simulink library "atlas_dynamic_library"  (Simulink 8.4)
settings: Solver=ode45  StartTime=0.0  StopTime=10.0  RelTol=1e-3
values from neighbouring files (symbols this model uses):
  atlas_arm_lr = lr    [atlas_joint_impctrl_sqrt_damping_test_settings_default.m]
  atlas_leg_lr = lr    [atlas_joint_impctrl_sqrt_damping_test_settings_default.m]
  B = d - 0.1*ones(NJL,1)    [atlas_joint_impctrl_sqrt_damping_test_settings_default.m]
  d = 0.2*ones(NJL,1)    [atlas_joint_impctrl_sqrt_damping_test_settings_default.m]
  muC = 8*ones(NJL,1)    [atlas_joint_impctrl_sqrt_damping_test_settings_default.m]
  q0 = q_l    [atlas_joint_impctrl_sqrt_damping_test_settings_default.m]
  qD0 = zeros(1,NJL)'    [atlas_joint_impctrl_sqrt_damping_test_settings_default.m]
  tau_c = muC - 4*ones(NJL,1)    [atlas_joint_impctrl_sqrt_damping_test_settings_default.m]
undefined symbols (not defined in the file or in its folder): atlas_version, delta_s, MPV, qD_s, tau_s
libraries: atlas_dynamic_library x28
settings Model: Creator=schappler  LastModifiedBy=vorndamme

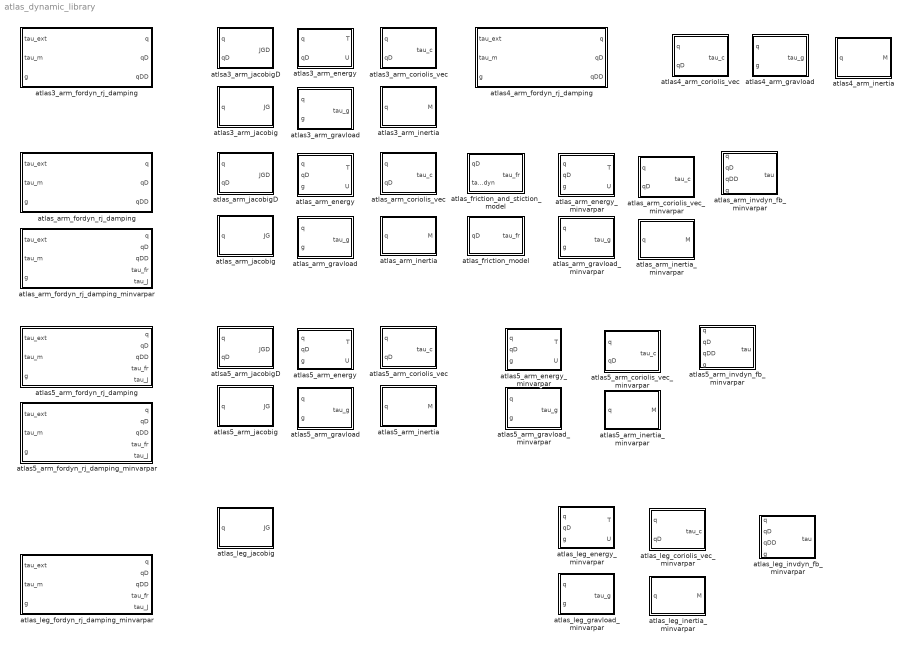
== system atlas_dynamic_library ==
  atlas3_arm_coriolis_vec : Subsystem  TreatAsAtomicUnit=on
  atlas3_arm_energy : Subsystem  TreatAsAtomicUnit=on
  atlas3_arm_fordyn_rj_damping : Subsystem  mask{q0=q0, qD0=qD0, d=d, muC=muC, atlas_arm_lr=atlas_arm_lr}
      mask prompts: q0 "q0 (initial pose)"; qD0 "qD0 (initial velocity)"; d "d (viscous friction)"; muC "muC (coulomb friction)"; atlas_arm_lr "atlas_arm_lr (Arm: left = true, right = false)"
  atlas3_arm_gravload : Subsystem  TreatAsAtomicUnit=on
  atlas3_arm_inertia : Subsystem  TreatAsAtomicUnit=on
  atlas3_arm_jacobig : Subsystem  TreatAsAtomicUnit=on
  atlas4_arm_coriolis_vec : Subsystem  TreatAsAtomicUnit=on
  atlas4_arm_fordyn_rj_damping : Subsystem  mask{q0=q0, qD0=qD0, d=d, muC=muC, atlas_arm_lr=atlas_arm_lr}
      mask prompts: q0 "q0 (initial pose)"; qD0 "qD0 (initial velocity)"; d "d (viscous friction)"; muC "muC (coulomb friction)"; atlas_arm_lr "atlas_arm_lr (Arm: left = true, right = false)"
  atlas4_arm_gravload : Subsystem  TreatAsAtomicUnit=on
  atlas4_arm_inertia : Subsystem  TreatAsAtomicUnit=on
  atlas5_arm_coriolis_vec : Subsystem  TreatAsAtomicUnit=on
  atlas5_arm_coriolis_vec_minvarpar : Subsystem  TreatAsAtomicUnit=on  mask{atlas_arm_lr=atlas_arm_lr, MPV=MPV}
      mask prompts: atlas_arm_lr "atlas_arm_lr (left = true, right = false)"; MPV "MPV (vector of minimal parameters)"
  atlas5_arm_energy : Subsystem  TreatAsAtomicUnit=on
  atlas5_arm_energy_minvarpar : Subsystem  TreatAsAtomicUnit=on  mask{MPV=MPV}
      mask prompts: MPV "MPV (vector of minimal parameters)"
  atlas5_arm_fordyn_rj_damping : Subsystem  mask{q0=q0, qD0=qD0, d=d, muC=muC, atlas_arm_lr=atlas_arm_lr}
      mask prompts: q0 "q0 (initial pose)"; qD0 "qD0 (initial velocity)"; d "d (viscous friction)"; muC "muC (coulomb friction)"; atlas_arm_lr "atlas_arm_lr (Arm: left = true, right = false)"
  atlas5_arm_fordyn_rj_damping_minvarpar : Subsystem  mask{q0=q0, qD0=qD0, d=d, muC=muC, atlas_arm_lr=atlas_arm_lr, MPV=MPV}
      mask prompts: q0 "q0 (initial pose)"; qD0 "qD0 (initial velocity)"; d "d (viscous friction)"; muC "muC (coulomb friction)"; atlas_arm_lr "atlas_arm_lr (Arm: left = true, right = false)"; MPV "MPV (minimal parameter vector)"
  atlas5_arm_gravload : Subsystem  TreatAsAtomicUnit=on
  atlas5_arm_gravload_minvarpar : Subsystem  TreatAsAtomicUnit=on  mask{atlas_arm_lr=atlas_arm_lr, MPV=MPV}
      mask prompts: atlas_arm_lr "atlas_arm_lr (left = true, right = false)"; MPV "MPV (vector of minimal parameters)"
  atlas5_arm_inertia : Subsystem  TreatAsAtomicUnit=on
  atlas5_arm_inertia_minvarpar : Subsystem  TreatAsAtomicUnit=on  mask{atlas_arm_lr=atlas_arm_lr, MPV=MPV}
      mask prompts: atlas_arm_lr "atlas_arm_lr (left = true, right = false)"; MPV "MPV (vector of minimal parameters)"
  atlas5_arm_invdyn_fb_minvarpar : Subsystem  TreatAsAtomicUnit=on  mask{MPV=MPV}
      mask prompts: MPV "MPV (vector of minimal parameters)"
  atlas5_arm_jacobig : Subsystem  TreatAsAtomicUnit=on
  atlas_arm_coriolis_vec : Subsystem  TreatAsAtomicUnit=on
  atlas_arm_coriolis_vec_minvarpar : Subsystem  TreatAsAtomicUnit=on  mask{atlas_arm_lr=atlas_arm_lr, atlas_version=atlas_version, MPV=MPV}
      mask prompts: atlas_arm_lr "atlas_arm_lr (left = true, right = false)"; atlas_version "atlas_version (3, 4)"; MPV "MPV (vecotr of minimal parameters)"
  atlas_arm_energy : Subsystem  TreatAsAtomicUnit=on
  atlas_arm_energy_minvarpar : Subsystem  TreatAsAtomicUnit=on  mask{MPV=MPV}
      mask prompts: MPV "MPV (vector of minimal parameters)"
  atlas_arm_fordyn_rj_damping : Subsystem  mask{q0=q0, qD0=qD0, d=d, muC=muC, atlas_arm_lr=atlas_arm_lr, atlas_version=atlas_version}
      mask prompts: q0 "q0 (initial pose)"; qD0 "qD0 (initial velocity)"; d "d (viscous friction)"; muC "muC (coulomb friction)"; atlas_arm_lr "atlas_arm_lr (Arm: left = true, right = false)"; atlas_version "atlas_version (3, 4)"
  atlas_arm_fordyn_rj_damping_minvarpar : Subsystem  mask{q0=q0, qD0=qD0, d=d, muC=muC, atlas_arm_lr=atlas_arm_lr, atlas_version=atlas_version, MPV=MPV}
      mask prompts: q0 "q0 (initial pose)"; qD0 "qD0 (initial velocity)"; d "d (viscous friction)"; muC "muC (coulomb friction)"; atlas_arm_lr "atlas_arm_lr (Arm: left = true, right = false)"; atlas_version "atlas_version (3, 4)"; MPV "MPV (minimal parameter vector)"
  atlas_arm_gravload : Subsystem  TreatAsAtomicUnit=on
  atlas_arm_gravload_minvarpar : Subsystem  TreatAsAtomicUnit=on  mask{atlas_arm_lr=atlas_arm_lr, atlas_version=atlas_version, MPV=MPV}
      mask prompts: atlas_arm_lr "atlas_arm_lr (left = true, right = false)"; atlas_version "atlas_version (3, 4)"; MPV "MPV (vector of minimal parameters)"
  atlas_arm_inertia : Subsystem  TreatAsAtomicUnit=on
  atlas_arm_inertia_minvarpar : Subsystem  TreatAsAtomicUnit=on  mask{atlas_arm_lr=atlas_arm_lr, atlas_version=atlas_version, MPV=MPV}
      mask prompts: atlas_arm_lr "atlas_arm_lr (left = true, right = false)"; atlas_version "atlas_version (3, 4)"; MPV "MPV (vector of minimal parameters)"
  atlas_arm_invdyn_fb_minvarpar : Subsystem  TreatAsAtomicUnit=on  mask{MPV=MPV}
      mask prompts: MPV "MPV (vector of minimal parameters)"
  atlas_arm_jacobig : Subsystem  TreatAsAtomicUnit=on
  atlas_arm_jacobigD : Subsystem  TreatAsAtomicUnit=on
  atlas_friction_and_stiction_model : Subsystem  TreatAsAtomicUnit=on  mask{tau_c=tau_c, B=B, tau_s=tau_s, qD_s=qD_s, delta_s=delta_s}
      mask prompts: tau_c "tau_c (vector with coulomb friciton momentums for all joints)"; B "B (vector with viscous friction coefficients of all joints)"; tau_s "tau_s (vector with sticition momentums of all joints)"; qD_s "qD_s (vector with Stribeck velocities of all joints)"; delta_s "delta_s (vector with stiction exponents for all joints)"
  atlas_friction_model : Subsystem  TreatAsAtomicUnit=on  mask{muC=muC, d=d}
  atlas_leg_coriolis_vec_minvarpar : Subsystem  TreatAsAtomicUnit=on  mask{atlas_arm_lr=atlas_leg_lr, atlas_version=atlas_version, MPV=MPV}
      mask prompts: atlas_arm_lr "atlas_arm_lr (left = true, right = false)"; atlas_version "atlas_version (3, 4)"; MPV "MPV (vecotr of minimal parameters)"
  atlas_leg_energy_minvarpar : Subsystem  TreatAsAtomicUnit=on  mask{MPV=MPV, atlas_version=atlas_version}
      mask prompts: MPV "MPV (vector of minimal parameters)"; atlas_version "Version"
  atlas_leg_fordyn_rj_damping_minvarpar : Subsystem  mask{q0=q0, qD0=qD0, d=d, muC=muC, atlas_arm_lr=atlas_leg_lr, atlas_version=uint8(5), MPV=MPV}
      mask prompts: q0 "q0 (initial pose)"; qD0 "qD0 (initial velocity)"; d "d (viscous friction)"; muC "muC (coulomb friction)"; atlas_arm_lr "atlas_leg_lr (Leg: left = true, right = false)"; atlas_version "atlas_version (3, 4)"; MPV "MPV (minimal parameter vector)"
  atlas_leg_gravload_minvarpar : Subsystem  TreatAsAtomicUnit=on  mask{atlas_arm_lr=atlas_leg_lr, atlas_version=atlas_version, MPV=MPV}
      mask prompts: atlas_arm_lr "atlas_arm_lr (left = true, right = false)"; atlas_version "atlas_version (3, 4)"; MPV "MPV (vector of minimal parameters)"
  atlas_leg_inertia_minvarpar : Subsystem  TreatAsAtomicUnit=on  mask{atlas_arm_lr=atlas_leg_lr, atlas_version=atlas_version, MPV=MPV}
      mask prompts: atlas_arm_lr "atlas_arm_lr (left = true, right = false)"; atlas_version "atlas_version (3, 4)"; MPV "MPV (vector of minimal parameters)"
  atlas_leg_invdyn_fb_minvarpar : Subsystem  TreatAsAtomicUnit=on  mask{MPV=MPV}
      mask prompts: MPV "MPV (vector of minimal parameters)"
  atlas_leg_jacobig : Subsystem  TreatAsAtomicUnit=on  mask{atlas_version=atlas_version, atlas_leg_lr=atlas_leg_lr}
      mask prompts: atlas_version "Version"; atlas_leg_lr "LeftRight"
  atlsa3_arm_jacobigD : Subsystem  TreatAsAtomicUnit=on
  atlsa5_arm_jacobigD : Subsystem  TreatAsAtomicUnit=on

== system atlas_dynamic_library/atlas3_arm_coriolis_vec ==
  q : Inport
  qD : Inport  Port=2
  mFcn_c : MATLAB Function  TreatAsAtomicUnit=on
  tau_c : Outport
  wires:
  mFcn_c/1(tau_c) -> tau_c/1
  qD/1 -> mFcn_c/2(qD)
  q/1 -> mFcn_c/1(q)

== system atlas_dynamic_library/atlas3_arm_energy ==
  q : Inport
  qD : Inport  Port=2
  atlas3_arm_energy_fb : MATLAB Function  TreatAsAtomicUnit=on  mask{edit_lr=atlas_arm_lr}
      mask prompts: edit_lr "Arm (left = true, right = false)"
      mask init:
      | if edit_lr == 1
      |   atlas_arm_lr = true; % left
      | else
      |   atlas_arm_lr = false; % right
      | end
  T : Outport
  U : Outport  Port=2
  wires:
  q/1 -> atlas3_arm_energy_fb/1(q)
  qD/1 -> atlas3_arm_energy_fb/2(qD)
  atlas3_arm_energy_fb/2(U) -> U/1
  atlas3_arm_energy_fb/1(T) -> T/1

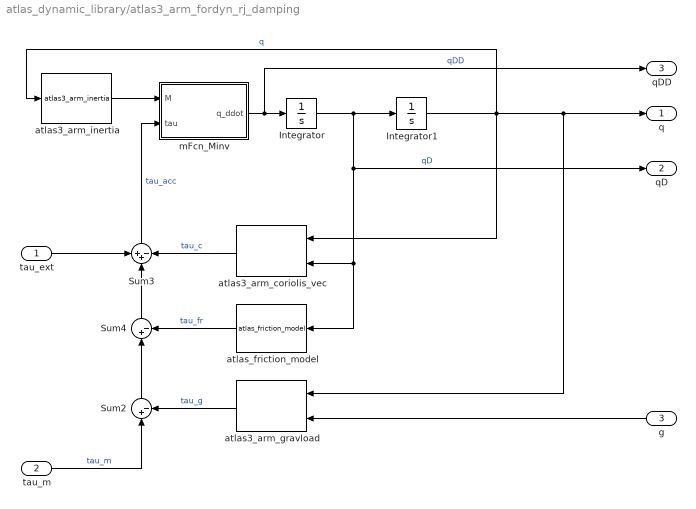
== system atlas_dynamic_library/atlas3_arm_fordyn_rj_damping ==
  "tau_ext " : Inport
  tau_m : Inport  Port=2
  g : Inport  Port=3
  Integrator : Integrator  InitialCondition=qD0
  Integrator1 : Integrator  InitialCondition=q0
  Sum2 : Sum  Inputs=|+-
  Sum3 : Sum  Inputs=++-
  Sum4 : Sum  Inputs=|+-
  atlas3_arm_coriolis_vec : atlas_dynamic_library/atlas3_arm_coriolis_vec
  atlas3_arm_gravload : atlas_dynamic_library/atlas3_arm_gravload
  atlas3_arm_inertia : atlas_dynamic_library/atlas3_arm_inertia
  atlas_friction_model : atlas_dynamic_library/atlas_friction_model  muC=muC  d=d
  mFcn_Minv : MATLAB Function  TreatAsAtomicUnit=on
  q : Outport
  qD : Outport  Port=2
  qDD : Outport  Port=3
  wires:
  atlas3_arm_gravload/1 -> Sum2/2  "tau_g"
  Integrator1/1 -> atlas3_arm_inertia/1, atlas3_arm_coriolis_vec/1, atlas3_arm_gravload/1, q/1  "q"
  Sum2/1 -> Sum4/1
  mFcn_Minv/1(q_ddot) -> qDD/1, Integrator/1  "qDD"
  Sum4/1 -> Sum3/2
  atlas3_arm_coriolis_vec/1 -> Sum3/3  "tau_c"
  atlas_friction_model/1 -> Sum4/2  "tau_fr"
  "tau_ext "/1 -> Sum3/1
  tau_m/1 -> Sum2/1  "tau_m"
  Integrator/1 -> qD/1, atlas_friction_model/1, atlas3_arm_coriolis_vec/2, Integrator1/1  "qD"
  Sum3/1 -> mFcn_Minv/2(tau)  "tau_acc"
  atlas3_arm_inertia/1 -> mFcn_Minv/1(M)
  g/1 -> atlas3_arm_gravload/2

== system atlas_dynamic_library/atlas3_arm_gravload ==
  q : Inport
  g : Inport  Port=2
  mFcn_g : MATLAB Function  TreatAsAtomicUnit=on
  tau_g : Outport
  wires:
  q/1 -> mFcn_g/1(q)
  mFcn_g/1(tau_g) -> tau_g/1
  g/1 -> mFcn_g/2(g)

== system atlas_dynamic_library/atlas3_arm_inertia ==
  q : Inport
  mFcn_M : MATLAB Function  TreatAsAtomicUnit=on
  M : Outport
  wires:
  q/1 -> mFcn_M/1(q)
  mFcn_M/1(M) -> M/1

== system atlas_dynamic_library/atlas3_arm_jacobig ==
  q : Inport
  atlas3_arm_jacobig : MATLAB Function  TreatAsAtomicUnit=on  mask{edit_lr=atlas_arm_lr}
      mask prompts: edit_lr "Arm (left = true, right = false)"
      mask init:
      | if edit_lr == 1
      |   atlas_arm_lr = true; % left
      | else
      |   atlas_arm_lr = false; % right
      | end
  JG : Outport
  wires:
  atlas3_arm_jacobig/1(JG) -> JG/1
  q/1 -> atlas3_arm_jacobig/1(q)

== system atlas_dynamic_library/atlas4_arm_coriolis_vec ==
  q : Inport
  qD : Inport  Port=2
  mFcn_c : MATLAB Function  TreatAsAtomicUnit=on
  tau_c : Outport
  wires:
  mFcn_c/1(tau_c) -> tau_c/1
  q/1 -> mFcn_c/1(q)
  qD/1 -> mFcn_c/2(qD)

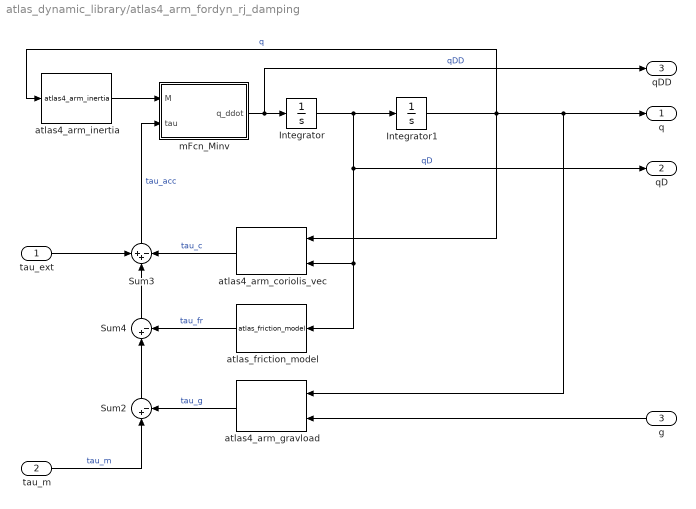
== system atlas_dynamic_library/atlas4_arm_fordyn_rj_damping ==
  "tau_ext " : Inport
  tau_m : Inport  Port=2
  g : Inport  Port=3
  Integrator : Integrator  InitialCondition=qD0
  Integrator1 : Integrator  InitialCondition=q0
  Sum2 : Sum  Inputs=|+-
  Sum3 : Sum  Inputs=++-
  Sum4 : Sum  Inputs=|+-
  atlas4_arm_coriolis_vec : atlas_dynamic_library/atlas4_arm_coriolis_vec
  atlas4_arm_gravload : atlas_dynamic_library/atlas4_arm_gravload
  atlas4_arm_inertia : atlas_dynamic_library/atlas4_arm_inertia
  atlas_friction_model : atlas_dynamic_library/atlas_friction_model  muC=muC  d=d
  mFcn_Minv : MATLAB Function  TreatAsAtomicUnit=on
  q : Outport
  qD : Outport  Port=2
  qDD : Outport  Port=3
  wires:
  atlas4_arm_gravload/1 -> Sum2/2  "tau_g"
  Integrator1/1 -> atlas4_arm_inertia/1, atlas4_arm_coriolis_vec/1, atlas4_arm_gravload/1, q/1  "q"
  Sum2/1 -> Sum4/1
  mFcn_Minv/1(q_ddot) -> qDD/1, Integrator/1  "qDD"
  Sum4/1 -> Sum3/2
  atlas4_arm_coriolis_vec/1 -> Sum3/3  "tau_c"
  atlas_friction_model/1 -> Sum4/2  "tau_fr"
  "tau_ext "/1 -> Sum3/1
  tau_m/1 -> Sum2/1  "tau_m"
  Integrator/1 -> qD/1, atlas_friction_model/1, atlas4_arm_coriolis_vec/2, Integrator1/1  "qD"
  Sum3/1 -> mFcn_Minv/2(tau)  "tau_acc"
  atlas4_arm_inertia/1 -> mFcn_Minv/1(M)
  g/1 -> atlas4_arm_gravload/2

== system atlas_dynamic_library/atlas4_arm_gravload ==
  q : Inport
  g : Inport  Port=2
  mFcn_g : MATLAB Function  TreatAsAtomicUnit=on
  tau_g : Outport
  wires:
  mFcn_g/1(tau_g) -> tau_g/1
  q/1 -> mFcn_g/1(q)
  g/1 -> mFcn_g/2(g)

== system atlas_dynamic_library/atlas4_arm_inertia ==
  q : Inport
  mFcn_M : MATLAB Function  TreatAsAtomicUnit=on
  M : Outport
  wires:
  q/1 -> mFcn_M/1(q)
  mFcn_M/1(M) -> M/1

== system atlas_dynamic_library/atlas5_arm_coriolis_vec ==
  q : Inport
  qD : Inport  Port=2
  mFcn_c : MATLAB Function  TreatAsAtomicUnit=on
  tau_c : Outport
  wires:
  mFcn_c/1(tau_c) -> tau_c/1
  qD/1 -> mFcn_c/2(qD)
  q/1 -> mFcn_c/1(q)

== system atlas_dynamic_library/atlas5_arm_coriolis_vec_minvarpar ==
  q : Inport
  qD : Inport  Port=2
  mFcn_c : MATLAB Function  TreatAsAtomicUnit=on
  tau_c : Outport
  wires:
  qD/1 -> mFcn_c/2(qD)
  q/1 -> mFcn_c/1(q)
  mFcn_c/1(tau_c) -> tau_c/1

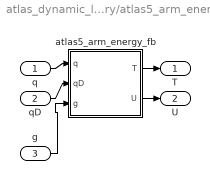
== system atlas_dynamic_library/atlas5_arm_energy ==
  q : Inport
  qD : Inport  Port=2
  g : Inport  Port=3
  atlas5_arm_energy_fb : MATLAB Function  TreatAsAtomicUnit=on  mask{edit_lr=atlas_arm_lr}
      mask prompts: edit_lr "Arm (left = true, right = false)"
      mask init:
      | if edit_lr == 1
      |   atlas_arm_lr = true; % left
      | else
      |   atlas_arm_lr = false; % right
      | end
  T : Outport
  U : Outport  Port=2
  wires:
  q/1 -> atlas5_arm_energy_fb/1(q)
  qD/1 -> atlas5_arm_energy_fb/2(qD)
  atlas5_arm_energy_fb/2(U) -> U/1
  atlas5_arm_energy_fb/1(T) -> T/1
  g/1 -> atlas5_arm_energy_fb/3(g)

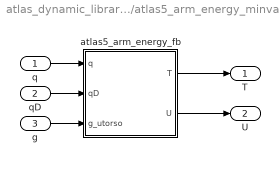
== system atlas_dynamic_library/atlas5_arm_energy_minvarpar ==
  q : Inport
  qD : Inport  Port=2
  g : Inport  Port=3
  atlas5_arm_energy_fb : MATLAB Function  TreatAsAtomicUnit=on
  T : Outport
  U : Outport  Port=2
  wires:
  g/1 -> atlas5_arm_energy_fb/3(g_utorso)
  q/1 -> atlas5_arm_energy_fb/1(q)
  atlas5_arm_energy_fb/2(U) -> U/1
  atlas5_arm_energy_fb/1(T) -> T/1
  qD/1 -> atlas5_arm_energy_fb/2(qD)

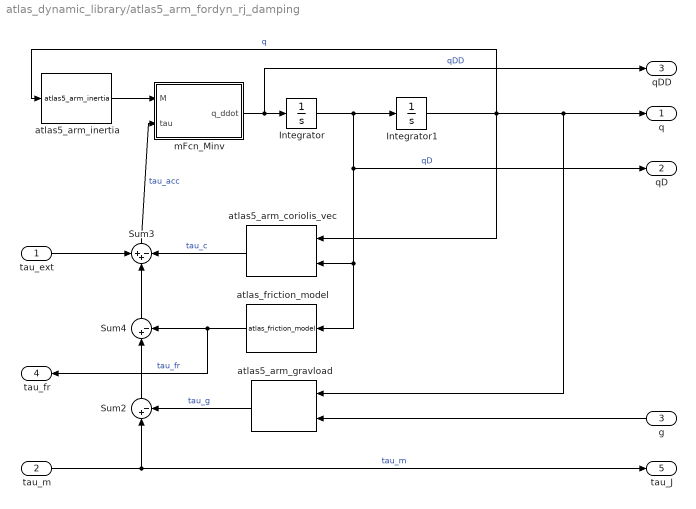
== system atlas_dynamic_library/atlas5_arm_fordyn_rj_damping ==
  "tau_ext " : Inport
  tau_m : Inport  Port=2
  g : Inport  Port=3
  Integrator : Integrator  InitialCondition=qD0
  Integrator1 : Integrator  InitialCondition=q0
  Sum2 : Sum  Inputs=|+-
  Sum3 : Sum  Inputs=++-
  Sum4 : Sum  Inputs=|+-
  atlas5_arm_coriolis_vec : atlas_dynamic_library/atlas5_arm_coriolis_vec
  atlas5_arm_gravload : atlas_dynamic_library/atlas5_arm_gravload
  atlas5_arm_inertia : atlas_dynamic_library/atlas5_arm_inertia
  atlas_friction_model : atlas_dynamic_library/atlas_friction_model  muC=muC  d=d
  mFcn_Minv : MATLAB Function  TreatAsAtomicUnit=on
  q : Outport
  qD : Outport  Port=2
  qDD : Outport  Port=3
  tau_fr : Outport  Port=4
  tau_J : Outport  Port=5
  wires:
  atlas5_arm_gravload/1 -> Sum2/2  "tau_g"
  Integrator1/1 -> atlas5_arm_inertia/1, atlas5_arm_coriolis_vec/1, atlas5_arm_gravload/1, q/1  "q"
  Sum2/1 -> Sum4/1
  mFcn_Minv/1(q_ddot) -> qDD/1, Integrator/1  "qDD"
  Sum4/1 -> Sum3/2
  atlas5_arm_coriolis_vec/1 -> Sum3/3  "tau_c"
  atlas_friction_model/1 -> tau_fr/1, Sum4/2  "tau_fr"
  "tau_ext "/1 -> Sum3/1
  Integrator/1 -> qD/1, atlas5_arm_coriolis_vec/2, atlas_friction_model/1, Integrator1/1  "qD"
  Sum3/1 -> mFcn_Minv/2(tau)  "tau_acc"
  atlas5_arm_inertia/1 -> mFcn_Minv/1(M)
  g/1 -> atlas5_arm_gravload/2
  tau_m/1 -> Sum2/1, tau_J/1  "tau_m"

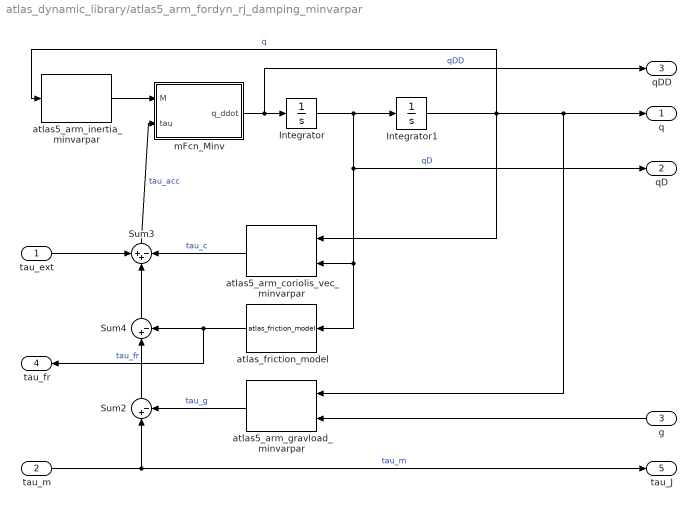
== system atlas_dynamic_library/atlas5_arm_fordyn_rj_damping_minvarpar ==
  "tau_ext " : Inport
  tau_m : Inport  Port=2
  g : Inport  Port=3
  Integrator : Integrator  InitialCondition=qD0
  Integrator1 : Integrator  InitialCondition=q0
  Sum2 : Sum  Inputs=|+-
  Sum3 : Sum  Inputs=++-
  Sum4 : Sum  Inputs=|+-
  atlas5_arm_coriolis_vec_minvarpar : atlas_dynamic_library/atlas5_arm_coriolis_vec_minvarpar
  atlas5_arm_gravload_minvarpar : atlas_dynamic_library/atlas5_arm_gravload_minvarpar
  atlas5_arm_inertia_minvarpar : atlas_dynamic_library/atlas5_arm_inertia_minvarpar
  atlas_friction_model : atlas_dynamic_library/atlas_friction_model  muC=muC  d=d
  mFcn_Minv : MATLAB Function  TreatAsAtomicUnit=on
  q : Outport
  qD : Outport  Port=2
  qDD : Outport  Port=3
  tau_fr : Outport  Port=4
  tau_J : Outport  Port=5
  wires:
  atlas5_arm_gravload_minvarpar/1 -> Sum2/2  "tau_g"
  Integrator1/1 -> atlas5_arm_coriolis_vec_minvarpar/1, atlas5_arm_inertia_minvarpar/1, atlas5_arm_gravload_minvarpar/1, q/1  "q"
  Sum2/1 -> Sum4/1
  mFcn_Minv/1(q_ddot) -> qDD/1, Integrator/1  "qDD"
  Sum4/1 -> Sum3/2
  atlas5_arm_coriolis_vec_minvarpar/1 -> Sum3/3  "tau_c"
  atlas_friction_model/1 -> tau_fr/1, Sum4/2  "tau_fr"
  "tau_ext "/1 -> Sum3/1
  Integrator/1 -> qD/1, atlas5_arm_coriolis_vec_minvarpar/2, atlas_friction_model/1, Integrator1/1  "qD"
  Sum3/1 -> mFcn_Minv/2(tau)  "tau_acc"
  atlas5_arm_inertia_minvarpar/1 -> mFcn_Minv/1(M)
  g/1 -> atlas5_arm_gravload_minvarpar/2
  tau_m/1 -> tau_J/1, Sum2/1  "tau_m"

== system atlas_dynamic_library/atlas5_arm_gravload ==
  q : Inport
  g : Inport  Port=2
  mFcn_g : MATLAB Function  TreatAsAtomicUnit=on
  tau_g : Outport
  wires:
  q/1 -> mFcn_g/1(q)
  mFcn_g/1(tau_g) -> tau_g/1
  g/1 -> mFcn_g/2(g)

== system atlas_dynamic_library/atlas5_arm_gravload_minvarpar ==
  q : Inport
  g : Inport  Port=2
  mFcn_g : MATLAB Function  TreatAsAtomicUnit=on
  tau_g : Outport
  wires:
  g/1 -> mFcn_g/2(g)
  mFcn_g/1(tau_g) -> tau_g/1
  q/1 -> mFcn_g/1(q)

== system atlas_dynamic_library/atlas5_arm_inertia ==
  q : Inport
  mFcn_M : MATLAB Function  TreatAsAtomicUnit=on
  M : Outport
  wires:
  q/1 -> mFcn_M/1(q)
  mFcn_M/1(M) -> M/1

== system atlas_dynamic_library/atlas5_arm_inertia_minvarpar ==
  q : Inport
  mFcn_M : MATLAB Function  TreatAsAtomicUnit=on
  M : Outport
  wires:
  mFcn_M/1(M) -> M/1
  q/1 -> mFcn_M/1(q)

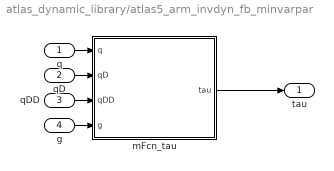
== system atlas_dynamic_library/atlas5_arm_invdyn_fb_minvarpar ==
  q : Inport
  qD : Inport  Port=2
  qDD : Inport  Port=3
  g : Inport  Port=4
  mFcn_tau : MATLAB Function  TreatAsAtomicUnit=on
  tau : Outport
  wires:
  g/1 -> mFcn_tau/4(g)
  qDD/1 -> mFcn_tau/3(qDD)
  qD/1 -> mFcn_tau/2(qD)
  q/1 -> mFcn_tau/1(q)
  mFcn_tau/1(tau) -> tau/1

== system atlas_dynamic_library/atlas5_arm_jacobig ==
  q : Inport
  atlas5_arm_jacobig : MATLAB Function  TreatAsAtomicUnit=on  mask{edit_lr=atlas_arm_lr}
      mask prompts: edit_lr "Arm (left = true, right = false)"
      mask init:
      | if edit_lr == 1
      |   atlas_arm_lr = true; % left
      | else
      |   atlas_arm_lr = false; % right
      | end
  JG : Outport
  wires:
  atlas5_arm_jacobig/1(JG) -> JG/1
  q/1 -> atlas5_arm_jacobig/1(q)

== system atlas_dynamic_library/atlas_arm_coriolis_vec ==
  q : Inport
  qD : Inport  Port=2
  mFcn_c : MATLAB Function  TreatAsAtomicUnit=on
  tau_c : Outport
  wires:
  mFcn_c/1(tau_c) -> tau_c/1
  q/1 -> mFcn_c/1(q)
  qD/1 -> mFcn_c/2(qD)

== system atlas_dynamic_library/atlas_arm_coriolis_vec_minvarpar ==
  q : Inport
  qD : Inport  Port=2
  mFcn_c : MATLAB Function  TreatAsAtomicUnit=on
  tau_c : Outport
  wires:
  qD/1 -> mFcn_c/2(qD)
  q/1 -> mFcn_c/1(q)
  mFcn_c/1(tau_c) -> tau_c/1

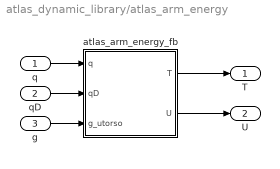
== system atlas_dynamic_library/atlas_arm_energy ==
  q : Inport
  qD : Inport  Port=2
  g : Inport  Port=3
  atlas_arm_energy_fb : MATLAB Function  TreatAsAtomicUnit=on
  T : Outport
  U : Outport  Port=2
  wires:
  qD/1 -> atlas_arm_energy_fb/2(qD)
  atlas_arm_energy_fb/1(T) -> T/1
  atlas_arm_energy_fb/2(U) -> U/1
  q/1 -> atlas_arm_energy_fb/1(q)
  g/1 -> atlas_arm_energy_fb/3(g_utorso)

== system atlas_dynamic_library/atlas_arm_energy_minvarpar ==
  q : Inport
  qD : Inport  Port=2
  g : Inport  Port=3
  atlas_arm_energy_fb : MATLAB Function  TreatAsAtomicUnit=on
  T : Outport
  U : Outport  Port=2
  wires:
  g/1 -> atlas_arm_energy_fb/3(g_utorso)
  q/1 -> atlas_arm_energy_fb/1(q)
  atlas_arm_energy_fb/2(U) -> U/1
  atlas_arm_energy_fb/1(T) -> T/1
  qD/1 -> atlas_arm_energy_fb/2(qD)

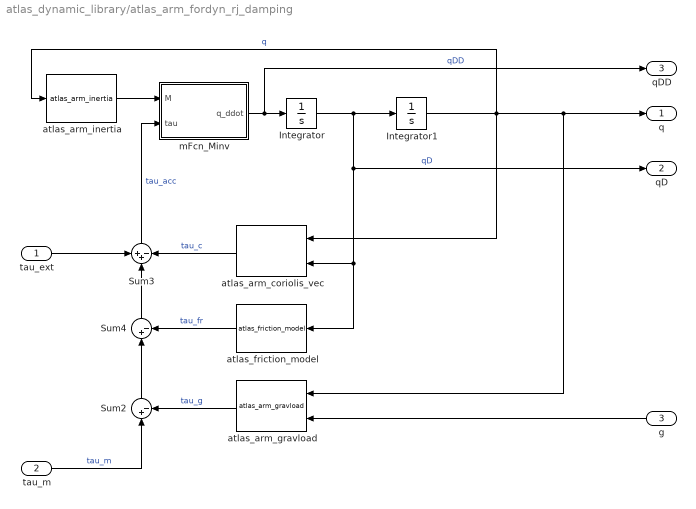
== system atlas_dynamic_library/atlas_arm_fordyn_rj_damping ==
  "tau_ext " : Inport
  tau_m : Inport  Port=2
  g : Inport  Port=3
  Integrator : Integrator  InitialCondition=qD0
  Integrator1 : Integrator  InitialCondition=q0
  Sum2 : Sum  Inputs=|+-
  Sum3 : Sum  Inputs=++-
  Sum4 : Sum  Inputs=|+-
  atlas_arm_coriolis_vec : atlas_dynamic_library/atlas_arm_coriolis_vec
  atlas_arm_gravload : atlas_dynamic_library/atlas_arm_gravload
  atlas_arm_inertia : atlas_dynamic_library/atlas_arm_inertia
  atlas_friction_model : atlas_dynamic_library/atlas_friction_model  muC=muC  d=d
  mFcn_Minv : MATLAB Function  TreatAsAtomicUnit=on
  q : Outport
  qD : Outport  Port=2
  qDD : Outport  Port=3
  wires:
  atlas_arm_gravload/1 -> Sum2/2  "tau_g"
  Integrator1/1 -> atlas_arm_inertia/1, atlas_arm_coriolis_vec/1, atlas_arm_gravload/1, q/1  "q"
  Sum2/1 -> Sum4/1
  mFcn_Minv/1(q_ddot) -> qDD/1, Integrator/1  "qDD"
  Sum4/1 -> Sum3/2
  atlas_arm_coriolis_vec/1 -> Sum3/3  "tau_c"
  atlas_friction_model/1 -> Sum4/2  "tau_fr"
  "tau_ext "/1 -> Sum3/1
  tau_m/1 -> Sum2/1  "tau_m"
  Integrator/1 -> qD/1, atlas_friction_model/1, atlas_arm_coriolis_vec/2, Integrator1/1  "qD"
  Sum3/1 -> mFcn_Minv/2(tau)  "tau_acc"
  atlas_arm_inertia/1 -> mFcn_Minv/1(M)
  g/1 -> atlas_arm_gravload/2

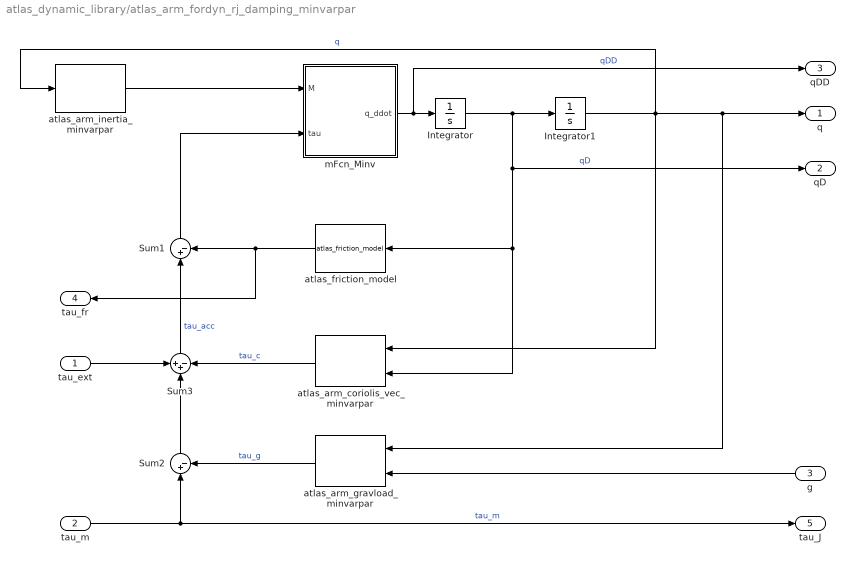
== system atlas_dynamic_library/atlas_arm_fordyn_rj_damping_minvarpar ==
  "tau_ext " : Inport
  tau_m : Inport  Port=2
  g : Inport  Port=3
  Integrator : Integrator  InitialCondition=qD0
  Integrator1 : Integrator  InitialCondition=q0
  Sum1 : Sum  Inputs=|+-
  Sum2 : Sum  Inputs=|+-
  Sum3 : Sum  Inputs=++-
  atlas_arm_coriolis_vec_minvarpar : atlas_dynamic_library/atlas_arm_coriolis_vec_minvarpar  atlas_arm_lr=atlas_arm_lr  atlas_version=atlas_version  MPV=MPV
  atlas_arm_gravload_minvarpar : atlas_dynamic_library/atlas_arm_gravload_minvarpar  atlas_arm_lr=atlas_arm_lr  atlas_version=atlas_version  MPV=MPV
  atlas_arm_inertia_minvarpar : atlas_dynamic_library/atlas_arm_inertia_minvarpar  atlas_arm_lr=atlas_arm_lr  atlas_version=atlas_version  MPV=MPV
  atlas_friction_model : atlas_dynamic_library/atlas_friction_model  muC=muC  d=d
  mFcn_Minv : MATLAB Function  TreatAsAtomicUnit=on
  q : Outport
  qD : Outport  Port=2
  qDD : Outport  Port=3
  tau_fr : Outport  Port=4
  tau_J : Outport  Port=5
  wires:
  atlas_arm_gravload_minvarpar/1 -> Sum2/2  "tau_g"
  Integrator1/1 -> atlas_arm_inertia_minvarpar/1, atlas_arm_coriolis_vec_minvarpar/1, atlas_arm_gravload_minvarpar/1, q/1  "q"
  mFcn_Minv/1(q_ddot) -> qDD/1, Integrator/1  "qDD"
  Sum2/1 -> Sum3/2
  atlas_arm_coriolis_vec_minvarpar/1 -> Sum3/3  "tau_c"
  "tau_ext "/1 -> Sum3/1
  tau_m/1 -> tau_J/1, Sum2/1  "tau_m"
  Integrator/1 -> qD/1, atlas_friction_model/1, atlas_arm_coriolis_vec_minvarpar/2, Integrator1/1  "qD"
  atlas_arm_inertia_minvarpar/1 -> mFcn_Minv/1(M)
  g/1 -> atlas_arm_gravload_minvarpar/2
  Sum3/1 -> Sum1/1  "tau_acc"
  atlas_friction_model/1 -> Sum1/2, tau_fr/1
  Sum1/1 -> mFcn_Minv/2(tau)

== system atlas_dynamic_library/atlas_arm_gravload ==
  q : Inport
  g : Inport  Port=2
  mFcn_g : MATLAB Function  TreatAsAtomicUnit=on
  tau_g : Outport
  wires:
  q/1 -> mFcn_g/1(q)
  mFcn_g/1(tau_g) -> tau_g/1
  g/1 -> mFcn_g/2(g)

== system atlas_dynamic_library/atlas_arm_gravload_minvarpar ==
  q : Inport
  g : Inport  Port=2
  mFcn_g : MATLAB Function  TreatAsAtomicUnit=on
  tau_g : Outport
  wires:
  g/1 -> mFcn_g/2(g)
  mFcn_g/1(tau_g) -> tau_g/1
  q/1 -> mFcn_g/1(q)

== system atlas_dynamic_library/atlas_arm_inertia ==
  q : Inport
  mFcn_M : MATLAB Function  TreatAsAtomicUnit=on
  M : Outport
  wires:
  mFcn_M/1(M) -> M/1
  q/1 -> mFcn_M/1(q)

== system atlas_dynamic_library/atlas_arm_inertia_minvarpar ==
  q : Inport
  mFcn_M : MATLAB Function  TreatAsAtomicUnit=on
  M : Outport
  wires:
  q/1 -> mFcn_M/1(q)
  mFcn_M/1(M) -> M/1

== system atlas_dynamic_library/atlas_arm_invdyn_fb_minvarpar ==
  q : Inport
  qD : Inport  Port=2
  qDD : Inport  Port=3
  g : Inport  Port=4
  mFcn_tau : MATLAB Function  TreatAsAtomicUnit=on
  tau : Outport
  wires:
  mFcn_tau/1(tau) -> tau/1
  q/1 -> mFcn_tau/1(q)
  qD/1 -> mFcn_tau/2(qD)
  qDD/1 -> mFcn_tau/3(qDD)
  g/1 -> mFcn_tau/4(g)

== system atlas_dynamic_library/atlas_arm_jacobig ==
  q : Inport
  atlas_arm_jacobig : MATLAB Function  TreatAsAtomicUnit=on  mask{edit_lr=atlas_arm_lr, edit_version=atlas_version}
      mask prompts: edit_lr "Arm (left = true, right = false)"; edit_version "Version (3, 4)"
      mask init:
      | if edit_lr == 1
      |   atlas_arm_lr = true; % left
      | else
      |   atlas_arm_lr = false; % right
      | end
      | 
      | if edit_version == 3
      |   atlas_version = uint8(3);
      | elseif edit_version == 4
      |   atlas_version = uint8(4);
      | else
      |   error('Version %d not implemented', edit_version);
      | end
  JG : Outport
  wires:
  q/1 -> atlas_arm_jacobig/1(q)
  atlas_arm_jacobig/1(JG) -> JG/1

== system atlas_dynamic_library/atlas_arm_jacobigD ==
  q : Inport
  qD : Inport  Port=2
  atlas_arm_jacobigD : MATLAB Function  TreatAsAtomicUnit=on  mask{edit_lr=atlas_arm_lr, edit_version=atlas_version}
      mask prompts: edit_lr "Arm (left = true, right = false)"; edit_version "Version (3, 4)"
      mask init:
      | if edit_lr == 1
      |   atlas_arm_lr = true; % left
      | else
      |   atlas_arm_lr = false; % right
      | end
  JGD : Outport
  wires:
  qD/1 -> atlas_arm_jacobigD/2(qD)
  q/1 -> atlas_arm_jacobigD/1(q)
  atlas_arm_jacobigD/1(JGD) -> JGD/1

== system atlas_dynamic_library/atlas_friction_and_stiction_model ==
  qD : Inport
  tau_dyn : Inport  Port=2
  atlas_friction_model : MATLAB Function  TreatAsAtomicUnit=on
  tau_fr : Outport
  wires:
  qD/1 -> atlas_friction_model/1(qD)
  atlas_friction_model/1(tau_reib) -> tau_fr/1
  tau_dyn/1 -> atlas_friction_model/2(tau_dyn)

== system atlas_dynamic_library/atlas_friction_model ==
  qD : Inport
  atlas_friction_model : MATLAB Function  TreatAsAtomicUnit=on
  tau_fr : Outport
  wires:
  qD/1 -> atlas_friction_model/1(qD)
  atlas_friction_model/1(tau_fr) -> tau_fr/1

== system atlas_dynamic_library/atlas_leg_coriolis_vec_minvarpar ==
  q : Inport
  qD : Inport  Port=2
  mFcn_c : MATLAB Function  TreatAsAtomicUnit=on
  tau_c : Outport
  wires:
  mFcn_c/1(tau_c) -> tau_c/1
  q/1 -> mFcn_c/1(q)
  qD/1 -> mFcn_c/2(qD)

== system atlas_dynamic_library/atlas_leg_energy_minvarpar ==
  q : Inport
  qD : Inport  Port=2
  g : Inport  Port=3
  atlas_leg_energy_fb : MATLAB Function  TreatAsAtomicUnit=on
  T : Outport
  U : Outport  Port=2
  wires:
  qD/1 -> atlas_leg_energy_fb/2(qD)
  atlas_leg_energy_fb/1(T) -> T/1
  atlas_leg_energy_fb/2(U) -> U/1
  q/1 -> atlas_leg_energy_fb/1(q)
  g/1 -> atlas_leg_energy_fb/3(g_utorso)

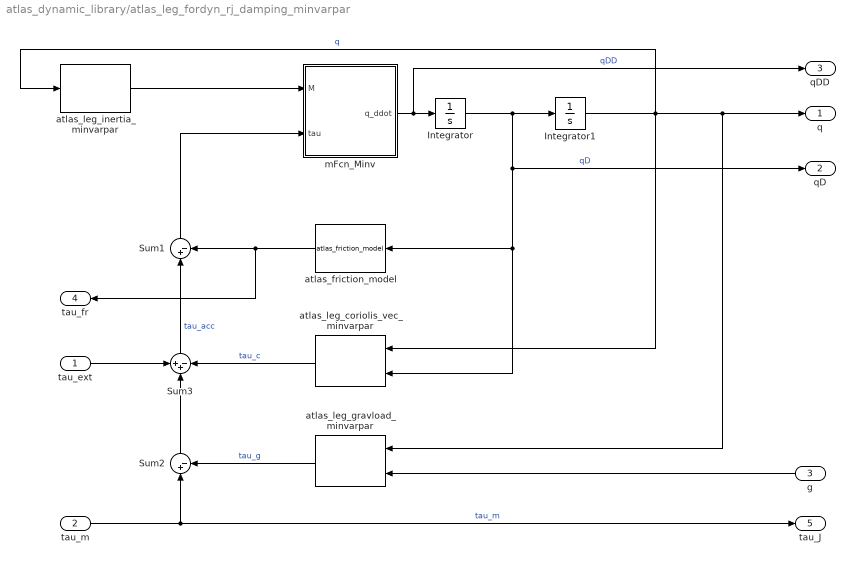
== system atlas_dynamic_library/atlas_leg_fordyn_rj_damping_minvarpar ==
  "tau_ext " : Inport
  tau_m : Inport  Port=2
  g : Inport  Port=3
  Integrator : Integrator  InitialCondition=qD0
  Integrator1 : Integrator  InitialCondition=q0
  Sum1 : Sum  Inputs=|+-
  Sum2 : Sum  Inputs=|+-
  Sum3 : Sum  Inputs=++-
  atlas_friction_model : atlas_dynamic_library/atlas_friction_model  muC=muC  d=d
  atlas_leg_coriolis_vec_minvarpar : atlas_dynamic_library/atlas_leg_coriolis_vec_minvarpar  atlas_arm_lr=atlas_leg_lr  atlas_version=atlas_version  MPV=MPV
  atlas_leg_gravload_minvarpar : atlas_dynamic_library/atlas_leg_gravload_minvarpar  atlas_arm_lr=atlas_leg_lr  atlas_version=atlas_version  MPV=MPV
  atlas_leg_inertia_minvarpar : atlas_dynamic_library/atlas_leg_inertia_minvarpar  atlas_arm_lr=atlas_leg_lr  atlas_version=atlas_version  MPV=MPV
  mFcn_Minv : MATLAB Function  TreatAsAtomicUnit=on
  q : Outport
  qD : Outport  Port=2
  qDD : Outport  Port=3
  tau_fr : Outport  Port=4
  tau_J : Outport  Port=5
  wires:
  Sum1/1 -> mFcn_Minv/2(tau)
  atlas_friction_model/1 -> tau_fr/1, Sum1/2
  Sum3/1 -> Sum1/1  "tau_acc"
  g/1 -> atlas_leg_gravload_minvarpar/2
  atlas_leg_inertia_minvarpar/1 -> mFcn_Minv/1(M)
  Integrator/1 -> Integrator1/1, atlas_leg_coriolis_vec_minvarpar/2, atlas_friction_model/1, qD/1  "qD"
  tau_m/1 -> Sum2/1, tau_J/1  "tau_m"
  "tau_ext "/1 -> Sum3/1
  atlas_leg_coriolis_vec_minvarpar/1 -> Sum3/3  "tau_c"
  Sum2/1 -> Sum3/2
  mFcn_Minv/1(q_ddot) -> Integrator/1, qDD/1  "qDD"
  Integrator1/1 -> atlas_leg_inertia_minvarpar/1, atlas_leg_coriolis_vec_minvarpar/1, atlas_leg_gravload_minvarpar/1, q/1  "q"
  atlas_leg_gravload_minvarpar/1 -> Sum2/2  "tau_g"

== system atlas_dynamic_library/atlas_leg_gravload_minvarpar ==
  q : Inport
  g : Inport  Port=2
  mFcn_g : MATLAB Function  TreatAsAtomicUnit=on
  tau_g : Outport
  wires:
  q/1 -> mFcn_g/1(q)
  mFcn_g/1(tau_g) -> tau_g/1
  g/1 -> mFcn_g/2(g)

== system atlas_dynamic_library/atlas_leg_inertia_minvarpar ==
  q : Inport
  mFcn_M : MATLAB Function  TreatAsAtomicUnit=on
  M : Outport
  wires:
  mFcn_M/1(M) -> M/1
  q/1 -> mFcn_M/1(q)

== system atlas_dynamic_library/atlas_leg_invdyn_fb_minvarpar ==
  q : Inport
  qD : Inport  Port=2
  qDD : Inport  Port=3
  g : Inport  Port=4
  mFcn_tau : MATLAB Function  TreatAsAtomicUnit=on
  tau : Outport
  wires:
  g/1 -> mFcn_tau/4(g)
  qDD/1 -> mFcn_tau/3(qDD)
  qD/1 -> mFcn_tau/2(qD)
  q/1 -> mFcn_tau/1(q)
  mFcn_tau/1(tau) -> tau/1

== system atlas_dynamic_library/atlas_leg_jacobig ==
  q : Inport
  atlas_leg_jacobig : MATLAB Function  TreatAsAtomicUnit=on  mask{edit_lr=atlas_leg_lr, atlas_version=atlas_version}
      mask prompts: edit_lr "Arm (left = true, right = false)"; atlas_version "Version"
      mask init:
      | if edit_lr == 1
      |   atlas_arm_lr = true; % left
      | else
      |   atlas_arm_lr = false; % right
      | end
  JG : Outport  PortDimensions=[6 6]
  wires:
  q/1 -> atlas_leg_jacobig/1(q)
  atlas_leg_jacobig/1(JG) -> JG/1

== system atlas_dynamic_library/atlsa3_arm_jacobigD ==
  q : Inport
  qD : Inport  Port=2
  atlas3_arm_jacobigD : MATLAB Function  TreatAsAtomicUnit=on  mask{edit_lr=atlas_arm_lr}
      mask prompts: edit_lr "Arm (left = true, right = false)"
      mask init:
      | if edit_lr == 1
      |   atlas_arm_lr = true; % left
      | else
      |   atlas_arm_lr = false; % right
      | end
  JGD : Outport
  wires:
  atlas3_arm_jacobigD/1(JGD) -> JGD/1
  qD/1 -> atlas3_arm_jacobigD/2(qD)
  q/1 -> atlas3_arm_jacobigD/1(q)

== system atlas_dynamic_library/atlsa5_arm_jacobigD ==
  q : Inport
  qD : Inport  Port=2
  atlas5_arm_jacobigD : MATLAB Function  TreatAsAtomicUnit=on  mask{edit_lr=atlas_arm_lr}
      mask prompts: edit_lr "Arm (left = true, right = false)"
      mask init:
      | if edit_lr == 1
      |   atlas_arm_lr = true; % left
      | else
      |   atlas_arm_lr = false; % right
      | end
  JGD : Outport
  wires:
  atlas5_arm_jacobigD/1(JGD) -> JGD/1
  qD/1 -> atlas5_arm_jacobigD/2(qD)
  q/1 -> atlas5_arm_jacobigD/1(q)

== matlab function atlas3_arm_fordyn_rj_damping/mFcn_Minv ==
  data: M input double; q_ddot output double; tau input double
function q_ddot = fcn(M,tau)
%#codegen
q_ddot=M\tau;

== matlab function atlas4_arm_inertia/mFcn_M ==
  data: q input double; M output double; atlas_arm_lr parameter double
function M = fcn(q, atlas_arm_lr)
%#codegen
M = atlas4_arm_inertia(q', atlas_arm_lr);

== matlab function atlas4_arm_coriolis_vec/mFcn_c ==
  data: q input double; qD input double; atlas_arm_lr parameter double; tau_c output double
function tau_c = fcn(q,qD, atlas_arm_lr)
%#codegen

tau_c=atlas4_arm_coriolisvec_fb(q', qD', atlas_arm_lr)';

== matlab function atlas4_arm_gravload/mFcn_g ==
  data: q input double; g input double; atlas_arm_lr parameter double; tau_g output double
function tau_g = fcn(q, g, atlas_arm_lr)
%#codegen

tau_g = atlas4_arm_gravload(q', g', atlas_arm_lr)';

== matlab function atlsa3_arm_jacobigD/atlas3_arm_jacobigD ==
  data: q input double; qD input double; JGD output double; atlas_arm_lr parameter double
function JGD = fcn(q, qD, atlas_arm_lr)
%#codegen

JGD = atlas3_arm_jacobigD(q', qD', atlas_arm_lr);

== matlab function atlas3_arm_energy/atlas3_arm_energy_fb ==
  data: q input double; qD input double; T output double; U output double; atlas_arm_lr parameter double
function [T, U] = fcn(q, qD, atlas_arm_lr)
%#codegen

T = atlas3_arm_energy_kinetic_fb_sym_lag(q', qD', atlas_arm_lr);

U = atlas3_arm_energy_potential_sym_lag(q', [0,0,-9.81], atlas_arm_lr);

== matlab function atlas3_arm_jacobig/atlas3_arm_jacobig ==
  data: q input double; JG output double; atlas_arm_lr parameter double
function JG = fcn(q, atlas_arm_lr)
%#codegen

JG = atlas3_arm_jacobig(q', atlas_arm_lr);

== matlab function atlas_arm_inertia/mFcn_M ==
  data: q input double; M output double; atlas_arm_lr parameter double; atlas_version parameter double
function M = fcn(q, atlas_arm_lr, atlas_version)
%#codegen
M = atlas_arm_inertia(q', atlas_arm_lr, atlas_version);

== matlab function atlas4_arm_fordyn_rj_damping/mFcn_Minv ==
  data: M input double; q_ddot output double; tau input double
function q_ddot = fcn(M,tau)
%#codegen
q_ddot=M\tau;

== matlab function atlas_arm_coriolis_vec/mFcn_c ==
  data: q input double; qD input double; atlas_arm_lr parameter double; tau_c output double; atlas_version parameter double
function tau_c = fcn(q,qD, atlas_arm_lr, atlas_version)
%#codegen

tau_c=atlas_arm_coriolisvec_fb(q', qD', atlas_arm_lr, atlas_version)';

== matlab function atlas_arm_gravload/mFcn_g ==
  data: q input double; g input double; atlas_arm_lr parameter double; tau_g output double; atlas_version parameter double
function tau_g = fcn(q, g, atlas_arm_lr, atlas_version)
%#codegen

tau_g = atlas_arm_gravload(q', g', atlas_arm_lr, atlas_version)';

== matlab function atlas_arm_gravload_minvarpar/mFcn_g ==
  data: q input double; g input double; MPV parameter double; atlas_arm_lr parameter double; tau_g output double; atlas_version parameter double
function tau_g = fcn(q, g, MPV, atlas_arm_lr, atlas_version)
%#codegen

tau_g = atlas_arm_gravload_plin_minpar_sym_lag_varpar( ...
  q', g', MPV, atlas_arm_lr, atlas_version)';

== matlab function atlas_arm_fordyn_rj_damping/mFcn_Minv ==
  data: M input double; q_ddot output double; tau input double
function q_ddot = fcn(M,tau)
%#codegen
q_ddot=M\tau;

== matlab function atlas_arm_inertia_minvarpar/mFcn_M ==
  data: q input double; MPV parameter double; M output double; atlas_arm_lr parameter double; atlas_version parameter double
function M = fcn(q, MPV, atlas_arm_lr, atlas_version)
%#codegen
M = atlas_arm_inertia_plin_minpar_sym_lag_varpar(q', MPV, atlas_arm_lr, atlas_version);

== matlab function atlas_arm_coriolis_vec_minvarpar/mFcn_c ==
  data: q input double; qD input double; MPV parameter double; atlas_arm_lr parameter double; tau_c output double; atlas_version parameter double
function tau_c = fcn(q,qD, MPV, atlas_arm_lr, atlas_version)
%#codegen

tau_c=atlas_arm_coriolisvec_fb_plin_minpar_sym_lag_varpar(q', qD', MPV, atlas_arm_lr, atlas_version)';

== matlab function atlas_arm_energy/atlas_arm_energy_fb ==
  data: q input double; qD input double; T output double; U output double; g_utorso input double; atlas_arm_lr parameter double; atlas_version parameter double
function [T, U] = fcn(q, qD, g_utorso, atlas_arm_lr, atlas_version)
%#codegen

T = atlas_arm_energy_kinetic_fb(q', qD', atlas_arm_lr, atlas_version);
U = atlas_arm_energy_potential(q', g_utorso', atlas_arm_lr, atlas_version);

== matlab function atlas_arm_jacobigD/atlas_arm_jacobigD ==
  data: q input double; qD input double; JGD output double; atlas_arm_lr parameter double; atlas_version parameter double
function JGD = fcn(q, qD, atlas_arm_lr, atlas_version)
%#codegen

JGD = atlas_arm_jacobigD(q', qD', atlas_arm_lr, atlas_version);

== matlab function atlas_arm_jacobig/atlas_arm_jacobig ==
  data: q input double; JG output double; atlas_arm_lr parameter double; atlas_version parameter double
function JG = fcn(q, atlas_arm_lr, atlas_version)
%#codegen

JG = atlas_arm_jacobig(q', atlas_arm_lr, atlas_version);

== matlab function atlas_arm_energy_minvarpar/atlas_arm_energy_fb ==
  data: q input double; qD input double; T output double; U output double; g_utorso input double; MPV parameter double; atlas_arm_lr parameter double; atlas_version parameter double
function [T, U] = fcn(q, qD, g_utorso, MPV, atlas_arm_lr, atlas_version)
%#codegen

T = atlas_arm_energy_kinetic_fb_minpar_sym_lag_varpar(q', qD', atlas_arm_lr, atlas_version);
U = atlas_arm_energy_potential_minpar_sym_lag_varpar(q', g_utorso', atlas_arm_lr, atlas_version);

== matlab function atlas3_arm_inertia/mFcn_M ==
  data: q input double; M output double; atlas_arm_lr parameter double
function M = fcn(q, atlas_arm_lr)
%#codegen
M = atlas3_arm_inertia(q', atlas_arm_lr);

== matlab function atlas3_arm_coriolis_vec/mFcn_c ==
  data: q input double; qD input double; atlas_arm_lr parameter double; tau_c output double
function tau_c = fcn(q,qD, atlas_arm_lr)
%#codegen

tau_c=atlas3_arm_coriolisvec_fb(q', qD', atlas_arm_lr)';

== matlab function atlas3_arm_gravload/mFcn_g ==
  data: q input double; g input double; atlas_arm_lr parameter double; tau_g output double
function tau_g = fcn(q, g, atlas_arm_lr)
%#codegen

tau_g = atlas3_arm_gravload(q', g', atlas_arm_lr)';

== matlab function atlas_arm_invdyn_fb_minvarpar/mFcn_tau ==
  data: q input double; qD input double; qDD input double; g input double; MPV parameter double; atlas_arm_lr parameter double; tau output double; atlas_version parameter double
function tau = fcn(q,qD, qDD, g, MPV, atlas_arm_lr, atlas_version)
%#codegen

tau=atlas_arm_invdyn_fb_plin_minpar_sym_lag_varpar(q', qD',qDD', g', MPV, atlas_arm_lr, atlas_version)';

== matlab function atlas_friction_model/atlas_friction_model ==
  data: qD input double; muC parameter double; tau_fr output double; d parameter double
function tau_fr = fcn(qD, muC, d)
%#codegen

tau_fr = ((atan(1000*qD)*(2/pi)) .* muC) + (qD .* d);

== matlab function atlas_arm_fordyn_rj_damping_minvarpar/mFcn_Minv ==
  data: M input double; q_ddot output double; tau input double
function q_ddot = fcn(M,tau)
%#codegen
q_ddot=M\tau;

== matlab function atlas_friction_and_stiction_model/atlas_friction_model ==
  data: qD input double; tau_dyn input double; tau_reib output double; tau_c parameter double; B parameter double; tau_s parameter double; qD_s parameter double; delta_s parameter double
function tau_reib = fcn(qD, tau_dyn, tau_c, B, tau_s, qD_s, delta_s)
%#codegen
tau_reib=zeros(length(qD),1);
for i=1:length(qD)
  if (abs(qD(i))<1e-9)
    if (abs(tau_dyn(i))<tau_s(i))
      tau_reib(i)=tau_dyn(i);
    else
      tau_reib(i)=tau_s(i)*sign(tau_dyn(i));
    end
  else
    tau_reib(i)=tau_c(i)*sign(qD(i)) + (tau_s(i)-tau_c(i))*exp(-abs(qD(i)/qD_s(i))^delta_s(i))*sign(qD(i)) + B(i)*qD(i);
  end
end

== matlab function atlas5_arm_energy/atlas5_arm_energy_fb ==
  data: q input double; qD input double; g input double; T output double; U output double; atlas_arm_lr parameter double
function [T, U] = fcn(q, qD, g, atlas_arm_lr)
%#codegen

T = atlas5_arm_energy_kinetic_fb_sym_lag(q', qD', atlas_arm_lr);

U = atlas5_arm_energy_potential_sym_lag(q', g', atlas_arm_lr);

== matlab function atlas5_arm_jacobig/atlas5_arm_jacobig ==
  data: q input double; JG output double; atlas_arm_lr parameter double
function JG = fcn(q, atlas_arm_lr)
%#codegen

JG = atlas5_arm_jacobig(q', atlas_arm_lr);

== matlab function atlas5_arm_gravload/mFcn_g ==
  data: q input double; g input double; atlas_arm_lr parameter double; tau_g output double
function tau_g = fcn(q, g, atlas_arm_lr)
%#codegen

tau_g = atlas5_arm_gravload(q', g', atlas_arm_lr)';

== matlab function atlas5_arm_coriolis_vec/mFcn_c ==
  data: q input double; qD input double; atlas_arm_lr parameter double; tau_c output double
function tau_c = fcn(q,qD, atlas_arm_lr)
%#codegen

tau_c=atlas5_arm_coriolisvec_fb(q', qD', atlas_arm_lr)';

== matlab function atlas5_arm_inertia/mFcn_M ==
  data: q input double; M output double; atlas_arm_lr parameter double
function M = fcn(q, atlas_arm_lr)
%#codegen
M = atlas5_arm_inertia(q', atlas_arm_lr);

== matlab function atlas5_arm_energy_minvarpar/atlas5_arm_energy_fb ==
  data: q input double; qD input double; T output double; U output double; g_utorso input double; MPV parameter double; atlas_arm_lr parameter double
function [T, U] = fcn(q, qD, g_utorso, MPV, atlas_arm_lr)
%#codegen

T = atlas5_arm_energy_kinetic_fb_plin_minpar_sym_lag_varpar(q', qD', MPV, atlas_arm_lr);
U = atlas5_arm_energy_potential_plin_minpar_sym_lag_varpar(q', g_utorso', MPV, atlas_arm_lr);

== matlab function atlas5_arm_gravload_minvarpar/mFcn_g ==
  data: q input double; g input double; MPV parameter double; atlas_arm_lr parameter double; tau_g output double
function tau_g = fcn(q, g, MPV, atlas_arm_lr)
%#codegen

tau_g = atlas5_arm_gravload_plin_minpar_sym_lag_varpar( ...
  q', g', MPV, atlas_arm_lr)';

== matlab function atlas5_arm_coriolis_vec_minvarpar/mFcn_c ==
  data: q input double; qD input double; MPV parameter double; atlas_arm_lr parameter double; tau_c output double
function tau_c = fcn(q,qD, MPV, atlas_arm_lr)
%#codegen

tau_c=atlas5_arm_coriolisvec_fb_plin_minpar_sym_lag_varpar(q', qD', MPV, atlas_arm_lr)';

== matlab function atlas5_arm_inertia_minvarpar/mFcn_M ==
  data: q input double; MPV parameter double; M output double; atlas_arm_lr parameter double
function M = fcn(q, MPV, atlas_arm_lr)
%#codegen
M = atlas5_arm_inertia_plin_minpar_sym_lag_varpar(q', MPV, atlas_arm_lr);

== matlab function atlas5_arm_invdyn_fb_minvarpar/mFcn_tau ==
  data: q input double; qD input double; qDD input double; g input double; MPV parameter double; atlas_arm_lr parameter double; tau output double
function tau = fcn(q,qD, qDD, g, MPV, atlas_arm_lr)
%#codegen

tau=atlas5_arm_invdyn_fb_plin_minpar_sym_lag_varpar(q', qD',qDD', g', MPV, atlas_arm_lr)';

== matlab function atlsa5_arm_jacobigD/atlas5_arm_jacobigD ==
  data: q input double; qD input double; JGD output double; atlas_arm_lr parameter double
function JGD = fcn(q, qD, atlas_arm_lr)
%#codegen

JGD = atlas5_arm_jacobigD(q', qD', atlas_arm_lr);

== matlab function atlas5_arm_fordyn_rj_damping/mFcn_Minv ==
  data: M input double; q_ddot output double; tau input double
function q_ddot = fcn(M,tau)
%#codegen
q_ddot=M\tau;

== matlab function atlas5_arm_fordyn_rj_damping_minvarpar/mFcn_Minv ==
  data: M input double; q_ddot output double; tau input double
function q_ddot = fcn(M,tau)
%#codegen
q_ddot=M\tau;

== matlab function atlas_leg_gravload_minvarpar/mFcn_g ==
  data: q input double; g input double; MPV parameter double; atlas_leg_lr parameter double; tau_g output double; atlas_version parameter double
function tau_g = fcn(q, g, MPV, atlas_leg_lr, atlas_version)
%#codegen

tau_g = atlas_leg_gravload_plin_minpar_sym_lag_varpar( ...
  q', g', MPV, atlas_leg_lr, atlas_version)';

== matlab function atlas_leg_inertia_minvarpar/mFcn_M ==
  data: q input double; MPV parameter double; M output double; atlas_leg_lr parameter double; atlas_version parameter double
function M = fcn(q, MPV, atlas_leg_lr, atlas_version)
%#codegen
M = atlas_leg_inertia_plin_minpar_sym_lag_varpar(q', MPV, atlas_leg_lr, atlas_version);

== matlab function atlas_leg_invdyn_fb_minvarpar/mFcn_tau ==
  data: q input double; qD input double; qDD input double; g input double; MPV parameter double; atlas_arm_lr parameter double; tau output double; atlas_version parameter double
function tau = fcn(q,qD, qDD, g, MPV, atlas_arm_lr, atlas_version)
%#codegen

tau=atlas_arm_invdyn_fb_plin_minpar_sym_lag_varpar(q', qD',qDD', g', MPV, atlas_arm_lr, atlas_version)';

== matlab function atlas_leg_coriolis_vec_minvarpar/mFcn_c ==
  data: q input double; qD input double; MPV parameter double; atlas_leg_lr parameter double; tau_c output double; atlas_version parameter double
function tau_c = fcn(q,qD, MPV, atlas_leg_lr, atlas_version)
%#codegen

tau_c=atlas_leg_coriolisvec_fb_plin_minpar_sym_lag_varpar(q', qD', MPV, atlas_leg_lr, atlas_version)';

== matlab function atlas_leg_energy_minvarpar/atlas_leg_energy_fb ==
  data: q input double; qD input double; T output double; U output double; g_utorso input double; MPV parameter double; atlas_leg_lr parameter double; atlas_version parameter double
function [T, U] = fcn(q, qD, g_utorso, MPV, atlas_leg_lr, atlas_version)
%#codegen

T = atlas_leg_energy_kinetic_fb_plin_minpar_varpar(q', qD', MPV, atlas_leg_lr, atlas_version);
U = atlas_leg_energy_potential_plin_minpar_varpar(q', g_utorso', MPV, atlas_leg_lr, atlas_version);

== matlab function atlas_leg_fordyn_rj_damping_minvarpar/mFcn_Minv ==
  data: M input double; q_ddot output double; tau input double
function q_ddot = fcn(M,tau)
%#codegen
q_ddot=M\tau;

== matlab function atlas_leg_jacobig/atlas_leg_jacobig ==
  data: q input double; JG output double; atlas_leg_lr parameter double; atlas_version parameter double
function JG = fcn(q, atlas_leg_lr, atlas_version)
%#codegen

JG = atlas_leg_jacobig(q', atlas_leg_lr, atlas_version);
